simulink model "Part_1"  (R2017b)
settings: Solver=VariableStepAuto  StartTime=0.0  StopTime=120  RelTol=1e-3
settings Model: Creator=Andrew Schueler  LastModifiedBy=Andrew Schueler

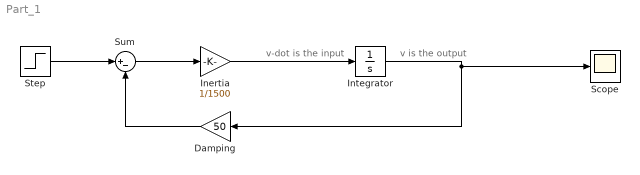
== system Part_1 ==
  note: v is the output
  note: v-dot is the input
  Damping : Gain  Gain=50
  "Inertia " : Gain  Gain=1/1500
  Integrator : Integrator
  Scope : Scope
  Step : Step  Time=0  After=500  SampleTime=0
  Sum : Sum  Inputs=|+-
  wires:
  "Inertia "/1 -> Integrator/1
  Integrator/1 -> Scope/1, Damping/1
  Sum/1 -> "Inertia "/1
  Damping/1 -> Sum/2
  Step/1 -> Sum/1
